simulink model "Figure_5_Fuel_Control_Block"  (R2021a)
settings: Solver=VariableStepAuto  StartTime=0.0  StopTime=10.0  RelTol=1e-3
model workspace (MAT data in the model file):
  K3 = Simulink.Parameter
  K3.Value = 2
  K3.DataType = 'auto'
  K3.Dimensions = [1 1]
  K6 = Simulink.Parameter
  K6.Value = 100
  K6.DataType = 'auto'
  K6.Dimensions = [1 1]
  T = Simulink.Parameter
  T.DataType = 'auto'
  T.Dimensions = [0 0]
  Tv = Simulink.Parameter
  Tv.DataType = 'auto'
  Tv.Dimensions = [0 0]
settings Model: Creator=Admin  LastModifiedBy=user

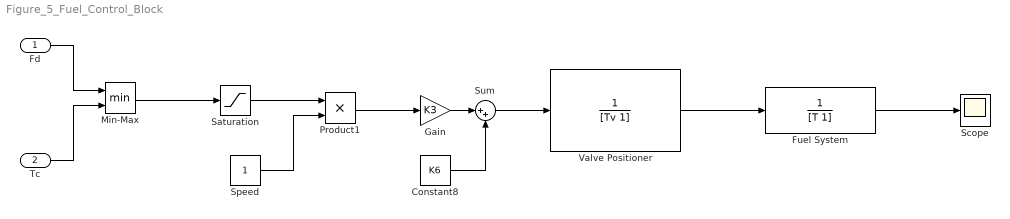
== system Figure_5_Fuel_Control_Block ==
  Fd : Inport
  Tc : Inport  Port=2
  " Gain " : Gain  Gain=K3
  " Saturation " : Saturate
  Constant8 : Constant  Value=K6
  Fuel System : TransferFcn  Denominator=[T 1]
  Min-Max : MinMax  Inputs=2
  Product1 : Product
  Scope : Scope
  Speed : Constant
  Sum : Sum  Inputs=|++
  Valve Positioner : TransferFcn  Denominator=[Tv 1]
  wires:
  Product1/1 -> " Gain "/1
  " Gain "/1 -> Sum/1
  Sum/1 -> Valve Positioner/1
  Valve Positioner/1 -> Fuel System/1
  Fuel System/1 -> Scope/1
  Speed/1 -> Product1/2
  " Saturation "/1 -> Product1/1
  Constant8/1 -> Sum/2
  Min-Max/1 -> " Saturation "/1
  Fd/1 -> Min-Max/1
  Tc/1 -> Min-Max/2
